simulink model "Grafica5"  (R2019a)
settings: Solver=VariableStepAuto  StartTime=0.0  StopTime=10.0  RelTol=1e-3
settings Model: Creator=rey_a  LastModifiedBy=rey_a

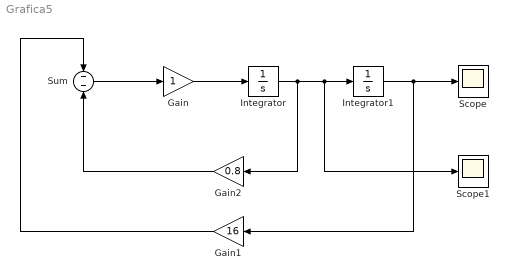
== system Grafica5 ==
  Gain : Gain
  Gain1 : Gain  Gain=16
  Gain2 : Gain  Gain=0.8
  Integrator : Integrator
  Integrator1 : Integrator  InitialCondition=2
  Scope : Scope
  Scope1 : Scope
  Sum : Sum  Inputs=--
  wires:
  Sum/1 -> Gain/1
  Gain/1 -> Integrator/1
  Gain2/1 -> Sum/2
  Gain1/1 -> Sum/1
  Integrator/1 -> Gain2/1, Integrator1/1, Scope1/1
  Integrator1/1 -> Gain1/1, Scope/1
